simulink model "sampleModel2077_3_sub_sub"  (R2023a)
settings: Solver=VariableStepAuto  StartTime=0.0  StopTime=10.0  RelTol=1e-3
libraries: hdlsllib x3, simulink x1
settings Model: Creator=user1  LastModifiedBy=user1

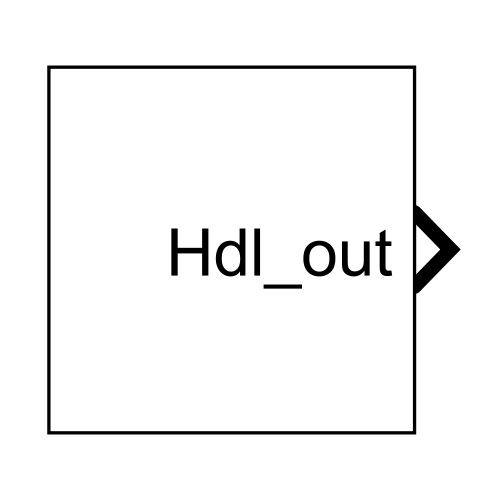
[thumbnail: Simulink's stored preview of the top-level diagram]
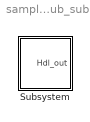
== system sampleModel2077_3_sub_sub ==
  Subsystem : Subsystem

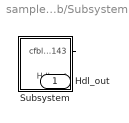
== system sampleModel2077_3_sub_sub/Subsystem ==
  Subsystem : Subsystem
  Hdl_out : Outport  OutDataTypeStr=uint8
  wires:
  Subsystem/1(cfblk143) -> Hdl_out/1

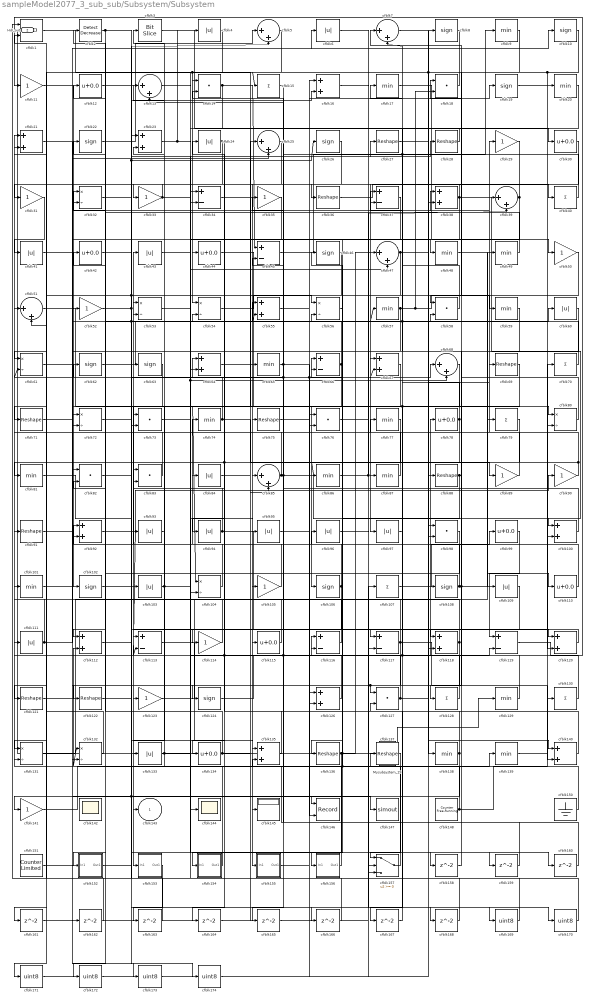
== system sampleModel2077_3_sub_sub/Subsystem/Subsystem ==
  Mysubsystem_19 : Subsystem  TreatAsAtomicUnit=on  RTWFcnName=Mysubsystem_19
      settings: RTWFcnNameOpts=User specified  RTWFileNameOpts=Use function name
  cfblk1 : Logic  AllPortsSameDT=off  OutDataTypeStr=boolean
  cfblk{8,10,19,22,26,46,62..63,102,106,108,124} (12 alike) : Signum
  cfblk{16,21,23,38,55,64,67,92,100,112,118,120,126,135,140} (15 alike) : Sum  OutDataTypeStr=uint8
  cfblk{9,17,20,48..49,57,59,65,74,77,81,86..87,101,129,138..139} (17 alike) : MinMax  OutDataTypeStr=uint8
  cfblk{4,6,24,41,43,60,84,93..97,103,109,111,133} (16 alike) : Abs  OutDataTypeStr=uint8  SaturateOnIntegerOverflow=off
  cfblk{32,53..54,56,61,72,80,104,131..132} (10 alike) : Product  Inputs=*/  OutDataTypeStr=uint8  RndMeth=Zero  SaturateOnIntegerOverflow=on
  cfblk{11,29,31,33,35,50,52,89..90,105,114,123,141} (13 alike) : Gain  OutDataTypeStr=uint8
  cfblk{15,40,70,79,107,128,130} (7 alike) : Sum  Inputs=+  OutDataTypeStr=uint8
  cfblk{12,30,42,44,78,99,110,115,134} (9 alike) : Bias  Bias=0.0  SaturateOnIntegerOverflow=off
  cfblk{34,37,45,66,113,116..117,119} (8 alike) : Sum  Inputs=+-  OutDataTypeStr=uint8
  cfblk{27..28,36,69,71,75,88,91,121..122,136..137} (12 alike) : Reshape
  cfblk{14,18,58,73,76,82..83,98,127} (9 alike) : DotProduct  OutDataTypeStr=uint8
  cfblk{5,7,13,25,39,47,51,68,85} (9 alike) : Sum  Inputs=|++  OutDataTypeStr=uint8
  cfblk142 : Scope
      settings: Floating=on
  cfblk144 : Scope
  cfblk145 : Display
  cfblk146 : Record  FileSettingsInternal="{\"entries\":[{\"content\":{\"excelSettings\":{\"content\":{},\"type\":\"Streamout.ExcelSettings\"}},\"type\":\"Streamout.FileSettingStorage\",\"uuid\":\"\"}],\"packageUris\":[\"http:\\/\\/schema.mathworks.com\\/mf0\\/streamout_blocks\\/R2020a\"],\"version\":\"1.0\"}"  Layout=[1 1]  SignalsInternal="{\"entries\":[{\"content\":{\"signals\":[{\"content\":{\"blockPath\":[],\"dimensions\":[1],\"domain\":\"\",\"lineColor\":\"#a2142f\",\"plots\":[1],\"port\":1,\"signalID\":61811,\"signalName\":\"cfblk39\"},\"type\":\"RecordBlkView.Signal\",\"uuid\":\"\"},{\"content\":{\"blockPath\":[],\"dimensions\":[1],\"domain\":\"\",\"lineColor\":\"#139fff\",\"plots\":[1],\"port\":2,\"signalID\":61814,\"signalName\":\"cfblk52\"},\"type\":\"RecordBlkView.Signal\",\"uuid\":\"\"}]},\"type\":\"RecordBlkView.InputSignals\",\"uuid\":\"\"}],\"packageUris\":[\"http:\\/\\/schema.mathworks.com\\/mf0\\/streamout_blocks\\/R2020a\"],\"version\":\"1.0\"}"  VisualizationBindings="{\"xyplotplugin\":{\"info\":[{\"series\":[{\"bindingParametersList\":[{\"parameter\":\"X-Axis\",\"signalID\":61811,\"signalName\":\"cfblk39\"},{\"parameter\":\"Y-Axis\",\"signalID\":61814,\"signalName\":\"cfblk52\"}],\"seriesID\":25996}],\"subplotID\":1}]}}"  CompatibilityTag=XY  st=-1
  cfblk147 : ToWorkspace  VariableName=simout  SaveFormat=Timeseries  SampleTime=-1
  cfblk148 : hdlsllib/Sources/Counter Free-Running  NumBits=16  tsamp=-1
  cfblk150 : Ground
  cfblk151 : hdlsllib/Sources/Counter Limited  uplimit=7  tsamp=-1
  cfblk152 : Subsystem
      settings: LibrarySourceBlock=|
      | hdlsllib/Ports &
      | Subsystems/Subsystem
  cfblk153 : Subsystem
      settings: LibrarySourceBlock=|
      | hdlsllib/Ports &
      | Subsystems/Subsystem
  cfblk154 : Subsystem
      settings: LibrarySourceBlock=|
      | hdlsllib/Ports &
      | Subsystems/Subsystem
  cfblk155 : Subsystem
      settings: LibrarySourceBlock=|
      | hdlsllib/Ports &
      | Subsystems/Subsystem
  cfblk156 : Subsystem
      settings: LibrarySourceBlock=|
      | hdlsllib/Ports &
      | Subsystems/Subsystem
  cfblk157 : Switch  OutDataTypeStr=uint8  SaturateOnIntegerOverflow=off  InputSameDT=off
  cfblk{158..168} (11 alike) : Delay  SampleTime=1
  cfblk{169..174} (6 alike) : DataTypeConversion  OutDataTypeStr=uint8  SaturateOnIntegerOverflow=off  RndMeth=Floor
  cfblk2 : simulink/Logic and Bit Operations/Detect Decrease  vinit=0.0  OutDataTypeStr=uint8
      settings: LibrarySourceBlock=|
      | hdlsllib/Logic and Bit
      | Operations/Detect
      | Decrease
  cfblk3 : hdlsllib/Logic and Bit Operations/Bit Slice  lidx=7  ridx=0
  cfblk143 : Outport  OutDataTypeStr=uint8  VectorParamsAs1DForOutWhenUnconnected=off
  Hdl_out : Outport  Port=2  OutDataTypeStr=uint8
  wires:
  Mysubsystem_19/1(Out1) -> cfblk129/1, Hdl_out/1
  cfblk174/1 -> cfblk98/2
  cfblk82/1 -> cfblk174/1
  cfblk173/1 -> cfblk98/1
  cfblk151/1 -> cfblk173/1
  cfblk172/1 -> cfblk107/1
  cfblk98/1 -> cfblk172/1
  cfblk171/1 -> cfblk76/2
  cfblk170/1 -> cfblk76/1
  cfblk122/1 -> cfblk170/1
  cfblk169/1 -> cfblk34/1
  cfblk76/1 -> cfblk169/1
  cfblk168/1 -> cfblk1/2
  cfblk167/1 -> cfblk127/2
  cfblk166/1 -> cfblk131/2
  cfblk32/1 -> cfblk166/1
  cfblk165/1 -> cfblk117/2
  cfblk164/1 -> cfblk126/2
  cfblk163/1 -> cfblk23/1
  cfblk153/1(Out1) -> cfblk163/1
  cfblk162/1 -> cfblk1/1
  cfblk41/1 -> cfblk162/1
  cfblk161/1 -> cfblk85/2
  cfblk160/1 -> cfblk135/2
  cfblk159/1 -> cfblk45/2
  cfblk13/1 -> cfblk159/1
  cfblk158/1 -> cfblk58/2
  cfblk72/1 -> cfblk158/1
  cfblk85/1 -> cfblk108/1, cfblk165/1, cfblk53/2
  cfblk118/1 -> cfblk124/1, cfblk83/2
  cfblk112/1 -> cfblk135/1
  cfblk21/1 -> cfblk82/1
  cfblk74/1 -> cfblk89/1, cfblk22/1
  cfblk102/1 -> cfblk68/1
  cfblk42/1 -> cfblk16/2, cfblk26/1
  cfblk75/1 -> cfblk16/1, cfblk67/2
  cfblk101/1 -> cfblk6/1
  cfblk154/1(Out1) -> cfblk23/2
  cfblk148/1 -> cfblk132/1, cfblk56/2, cfblk130/1
  cfblk78/1 -> cfblk164/1, cfblk171/1, cfblk37/2
  cfblk115/1 -> cfblk83/1
  cfblk70/1 -> cfblk32/2
  cfblk129/1 -> cfblk66/2, cfblk77/1
  cfblk26/1 -> cfblk71/1
  cfblk18/1 -> cfblk14/1
  cfblk157/1 -> cfblk21/2
  cfblk100/1 -> cfblk61/2, cfblk14/2
  cfblk155/1(Out1) -> cfblk137/1
  cfblk117/1 -> cfblk127/1, cfblk132/2, cfblk140/2, cfblk82/2
  cfblk152/1(Out1) -> cfblk5/2, cfblk55/2
  cfblk9/1 -> cfblk58/1
  cfblk103/1 -> cfblk144/1, cfblk13/1
  cfblk2/1 -> cfblk122/1, cfblk118/2
  cfblk96/1 -> cfblk157/3
  cfblk73/1 -> cfblk27/1
  cfblk20/1 -> cfblk67/1
  cfblk86/1 -> cfblk39/2, cfblk160/1
  cfblk52/1 -> cfblk146/2, cfblk168/1, cfblk28/1
  cfblk64/1 -> cfblk80/2
  cfblk91/1 -> cfblk39/1
  cfblk108/1 -> cfblk18/1, cfblk110/1, cfblk64/1
  cfblk150/1 -> cfblk112/2
  cfblk24/1 -> cfblk114/1, cfblk92/2
  cfblk126/1 -> cfblk113/2, cfblk84/1
  cfblk66/1 -> cfblk123/1, cfblk42/1
  cfblk84/1 -> cfblk66/1
  cfblk124/1 -> cfblk116/1
  cfblk27/1 -> cfblk138/1
  cfblk133/1 -> cfblk53/1, cfblk119/2
  cfblk48/1 -> cfblk109/1
  cfblk138/1 -> cfblk46/1, cfblk161/1
  cfblk6/1 -> cfblk157/2
  cfblk109/1 -> cfblk117/1
  cfblk60/1 -> cfblk152/1(In1)
  cfblk88/1 -> cfblk136/1, cfblk118/1
  cfblk97/1 -> cfblk37/1, cfblk57/1
  cfblk12/1 -> cfblk10/1
  cfblk95/1 -> cfblk126/1
  cfblk7/1 -> cfblk140/1
  cfblk81/1 -> cfblk103/1
  cfblk130/1 -> cfblk111/1
  cfblk79/1 -> cfblk113/1
  cfblk59/1 -> cfblk128/1
  cfblk8/1 -> cfblk15/1, cfblk38/2
  cfblk116/1 -> cfblk101/1
  cfblk19/1 -> cfblk20/1
  cfblk36/1 -> cfblk40/1
  cfblk3/1 -> cfblk88/1
  cfblk35/1 -> cfblk52/1
  cfblk61/1 -> cfblk143/1
  cfblk77/1 -> cfblk121/1
  cfblk62/1 -> cfblk55/1
  cfblk110/1 -> cfblk96/1
  cfblk136/1 -> cfblk116/2, cfblk47/1, cfblk154/1(In1)
  cfblk50/1 -> cfblk112/1, cfblk73/2
  cfblk65/1 -> cfblk105/1, cfblk147/1
  cfblk23/1 -> cfblk95/1, cfblk68/2, cfblk4/1
  cfblk114/1 -> cfblk92/1
  cfblk46/1 -> cfblk81/1
  cfblk93/1 -> cfblk3/1
  cfblk1/1 -> cfblk65/1
  cfblk53/1 -> cfblk38/1
  cfblk30/1 -> cfblk87/1
  cfblk67/1 -> cfblk94/1
  cfblk16/1 -> cfblk30/1
  cfblk141/1 -> cfblk139/1
  cfblk134/1 -> cfblk25/1, cfblk2/1
  cfblk57/1 -> cfblk59/1, cfblk18/2, cfblk72/2
  cfblk10/1 -> cfblk120/2, cfblk141/1
  cfblk40/1 -> cfblk7/2, cfblk13/2
  cfblk58/1 -> cfblk17/1
  cfblk139/1 -> cfblk70/1
  cfblk29/1 -> cfblk61/1
  cfblk55/1 -> cfblk19/1
  cfblk140/1 -> cfblk54/2
  cfblk14/1 -> cfblk45/1, cfblk34/2
  cfblk123/1 -> cfblk8/1
  cfblk71/1 -> cfblk60/1
  cfblk89/1 -> cfblk62/1
  cfblk127/1 -> cfblk93/1, cfblk35/1, cfblk69/1
  cfblk56/1 -> cfblk156/1(In1)
  cfblk47/1 -> cfblk97/1, cfblk100/2
  cfblk15/1 -> cfblk85/1
  cfblk113/1 -> cfblk145/1
  cfblk121/1 -> cfblk79/1
  cfblk37/1 -> cfblk134/1
  cfblk49/1 -> cfblk12/1
  cfblk51/1 -> cfblk80/1
  cfblk135/1 -> cfblk24/1
  cfblk43/1 -> cfblk48/1
  cfblk4/1 -> cfblk44/1, cfblk104/2
  cfblk106/1 -> cfblk32/1, cfblk133/1
  cfblk87/1 -> cfblk73/1
  cfblk5/1 -> cfblk131/1
  cfblk39/1 -> cfblk36/1, cfblk146/1
  cfblk63/1 -> cfblk153/1(In1)
  cfblk80/1 -> cfblk7/1
  cfblk132/1 -> cfblk51/2
  cfblk99/1 -> cfblk119/1
  cfblk54/1 -> cfblk56/1
  cfblk44/1 -> cfblk106/1
  cfblk31/1 -> cfblk41/1
  cfblk128/1 -> cfblk78/1
  cfblk11/1 -> cfblk72/1
  cfblk17/1 -> cfblk50/1
  cfblk119/1 -> cfblk11/1
  cfblk45/1 -> cfblk9/1
  cfblk83/1 -> cfblk51/1
  cfblk28/1 -> cfblk54/1
  cfblk25/1 -> cfblk75/1
  cfblk105/1 -> cfblk43/1
  cfblk131/1 -> cfblk49/1
  cfblk104/1 -> cfblk74/1
  cfblk90/1 -> cfblk29/1, cfblk86/1
  cfblk111/1 -> cfblk91/1, cfblk25/2
  cfblk38/1 -> cfblk100/1, cfblk64/2, cfblk33/1
  cfblk22/1 -> cfblk5/1
  cfblk120/1 -> cfblk115/1
  cfblk33/1 -> cfblk31/1, cfblk47/2
  cfblk69/1 -> cfblk102/1
  cfblk137/1 -> cfblk157/1
  cfblk92/1 -> cfblk90/1
  cfblk34/1 -> cfblk155/1(In1)
  cfblk68/1 -> cfblk104/1, cfblk167/1
  cfblk94/1 -> cfblk120/1, cfblk63/1
  cfblk107/1 -> cfblk99/1
  cfblk156/1(Out1) -> cfblk21/1

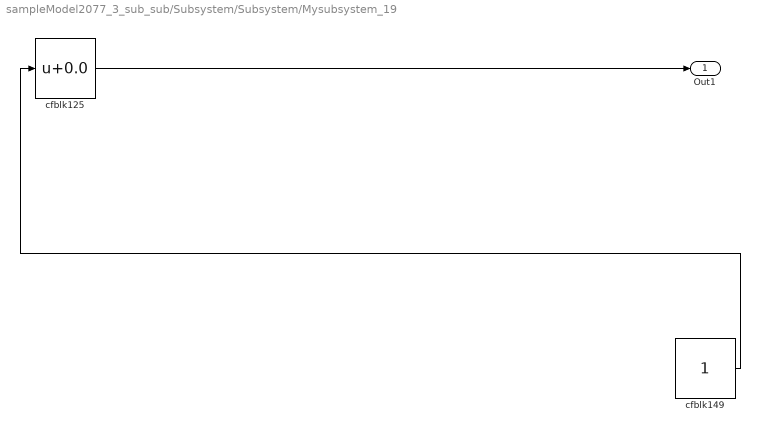
== system sampleModel2077_3_sub_sub/Subsystem/Subsystem/Mysubsystem_19 ==
  cfblk125 : Bias  Bias=0.0  SaturateOnIntegerOverflow=off
  cfblk149 : Constant  SampleTime=-1
  Out1 : Outport
  wires:
  cfblk149/1 -> cfblk125/1
  cfblk125/1 -> Out1/1

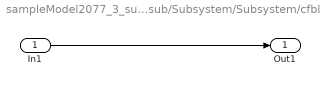
== system sampleModel2077_3_sub_sub/Subsystem/Subsystem/cfblk152 ==
  In1 : Inport
  Out1 : Outport
  wires:
  In1/1 -> Out1/1

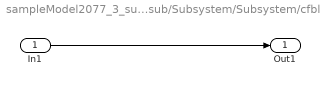
== system sampleModel2077_3_sub_sub/Subsystem/Subsystem/cfblk153 ==
  In1 : Inport
  Out1 : Outport
  wires:
  In1/1 -> Out1/1

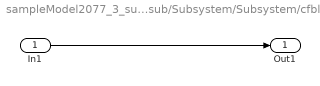
== system sampleModel2077_3_sub_sub/Subsystem/Subsystem/cfblk154 ==
  In1 : Inport
  Out1 : Outport
  wires:
  In1/1 -> Out1/1

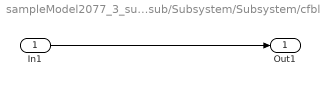
== system sampleModel2077_3_sub_sub/Subsystem/Subsystem/cfblk155 ==
  In1 : Inport
  Out1 : Outport
  wires:
  In1/1 -> Out1/1

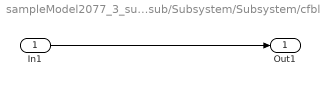
== system sampleModel2077_3_sub_sub/Subsystem/Subsystem/cfblk156 ==
  In1 : Inport
  Out1 : Outport
  wires:
  In1/1 -> Out1/1
